simulink model "Ecotron"  (R2019b)
settings: Solver=FixedStepAuto  StartTime=0.0  StopTime=1  FixedStep=0.001  RelTol=1e-3  EnableMultiTasking=on
InitFcn:
  | EcoCoder_PreCheckLic();
libraries: CoderSF_BSW_Libs x228, SF_CanService_Libs x49, simulink x33, dspstat3 x6
(part 4 of 6)

== system Ecotron/Input/By-wire/PDS/Subsystem2 ==
  Bus Creator4 : BusCreator  Inputs=5
  Bus Creator5 : BusCreator  Inputs=4  OutDataTypeStr=Bus: Msg
      settings: InheritFromInputs=off
  Read CAN Message3 : SF_CanService_Libs/Read CAN Message  typeCAN=Connected  channel=CAN_C  mEn=off  msgInfo=ld_pds  msgItermStore=PDS_Current2Master  msgIterm=PDS_Current2Master  valid=on  stale=on  motoBit=off  setSignalName=on  flgCustomMonitorVariableRules=on  defineSignalName=off  prefixSignal='rx'  flgValTest=off  flgNoFixed=on  tSample=Task_L1ms  modeCode=Parameterless
  Subsystem1 : Subsystem
  Write and Read Measurement : CoderSF_BSW_Libs/Calibration & Measurement/Write and Read Measurement  variable_name=PDS_CH5Current  variable_value=0  variable_type=single  numD=1  unitStr=""  descStr=""
      settings: AttributesFormatString=type:%<variable_type> Dimensions:%<numD>  SourceProductName=EcoCoder Blocks
  Write and Read Measurement1 : CoderSF_BSW_Libs/Calibration & Measurement/Write and Read Measurement  variable_name=PDS_CH6Current  variable_value=0  variable_type=single  numD=1  unitStr=""  descStr=""
      settings: AttributesFormatString=type:%<variable_type> Dimensions:%<numD>  SourceProductName=EcoCoder Blocks
  Write and Read Measurement2 : CoderSF_BSW_Libs/Calibration & Measurement/Write and Read Measurement  variable_name=PDS_CH7Current  variable_value=0  variable_type=single  numD=1  unitStr=""  descStr=""
      settings: AttributesFormatString=type:%<variable_type> Dimensions:%<numD>  SourceProductName=EcoCoder Blocks
  Write and Read Measurement3 : CoderSF_BSW_Libs/Calibration & Measurement/Write and Read Measurement  variable_name=PDS_CH8Current  variable_value=0  variable_type=single  numD=1  unitStr=""  descStr=""
      settings: AttributesFormatString=type:%<variable_type> Dimensions:%<numD>  SourceProductName=EcoCoder Blocks
  Current2 : Outport
  wires:
  Read CAN Message3/2 -> Subsystem1/2(Msg_cnt)
  Read CAN Message3/1 -> Subsystem1/1("Available_in ")
  Bus Creator5/1 -> Bus Creator4/1  "Msg"
  Read CAN Message3/4 -> Write and Read Measurement1/1  "rxCURRENT6"
  Subsystem1/4(Msg_Freq) -> Bus Creator5/4  "Freq"
  Subsystem1/1("Available ") -> Bus Creator5/1  "Available"
  Subsystem1/3(Timeout_Err) -> Bus Creator5/3  "Timeout"
  Subsystem1/2(Cnt) -> Bus Creator5/2  "Cnt"
  Read CAN Message3/3 -> Write and Read Measurement/1  "rxCURRENT5"
  Read CAN Message3/6 -> Write and Read Measurement3/1  "rxCURRENT8"
  Read CAN Message3/5 -> Write and Read Measurement2/1  "rxCURRENT7"
  Bus Creator4/1 -> Current2/1  "Current2"
  Write and Read Measurement/1 -> Bus Creator4/2  "PDS_CH5Current"
  Write and Read Measurement1/1 -> Bus Creator4/3  "PDS_CH6Current"
  Write and Read Measurement2/1 -> Bus Creator4/4  "PDS_CH7Current"
  Write and Read Measurement3/1 -> Bus Creator4/5  "PDS_CH8Current"

== system Ecotron/Input/By-wire/PDS/Subsystem3 ==
  Bus Creator10 : BusCreator  Inputs=5
  Bus Creator3 : BusCreator  Inputs=4  OutDataTypeStr=Bus: Msg
      settings: InheritFromInputs=off
  Read CAN Message2 : SF_CanService_Libs/Read CAN Message  typeCAN=Connected  channel=CAN_C  mEn=off  msgInfo=ld_pds  msgItermStore=PDS_Current1Master  msgIterm=PDS_Current1Master  valid=on  stale=on  motoBit=off  setSignalName=on  flgCustomMonitorVariableRules=on  defineSignalName=off  prefixSignal='rx'  flgValTest=off  flgNoFixed=on  tSample=Task_L1ms  modeCode=Parameterless
  Subsystem2 : Subsystem
  Write and Read Measurement : CoderSF_BSW_Libs/Calibration & Measurement/Write and Read Measurement  variable_name=PDS_CH1Current  variable_value=0  variable_type=single  numD=1  unitStr=""  descStr=""
      settings: AttributesFormatString=type:%<variable_type> Dimensions:%<numD>  SourceProductName=EcoCoder Blocks
  Write and Read Measurement1 : CoderSF_BSW_Libs/Calibration & Measurement/Write and Read Measurement  variable_name=PDS_CH2Current  variable_value=0  variable_type=single  numD=1  unitStr=""  descStr=""
      settings: AttributesFormatString=type:%<variable_type> Dimensions:%<numD>  SourceProductName=EcoCoder Blocks
  Write and Read Measurement2 : CoderSF_BSW_Libs/Calibration & Measurement/Write and Read Measurement  variable_name=PDS_CH3Current  variable_value=0  variable_type=single  numD=1  unitStr=""  descStr=""
      settings: AttributesFormatString=type:%<variable_type> Dimensions:%<numD>  SourceProductName=EcoCoder Blocks
  Write and Read Measurement3 : CoderSF_BSW_Libs/Calibration & Measurement/Write and Read Measurement  variable_name=PDS_CH4Current  variable_value=0  variable_type=single  numD=1  unitStr=""  descStr=""
      settings: AttributesFormatString=type:%<variable_type> Dimensions:%<numD>  SourceProductName=EcoCoder Blocks
  Current1 : Outport
  wires:
  Subsystem2/4(Msg_Freq) -> Bus Creator3/4  "MsgFreq"
  Read CAN Message2/1 -> Subsystem2/1("Available_in ")
  Subsystem2/1("Available ") -> Bus Creator3/1  "Available"
  Subsystem2/3(Timeout_Err) -> Bus Creator3/3  "Timeout"
  Bus Creator3/1 -> Bus Creator10/1  "Msg"
  Read CAN Message2/2 -> Subsystem2/2(Msg_cnt)
  Subsystem2/2(Cnt) -> Bus Creator3/2  "Cnt"
  Read CAN Message2/5 -> Write and Read Measurement2/1  "rxCURRENT3"
  Read CAN Message2/4 -> Write and Read Measurement1/1  "rxCURRENT2"
  Read CAN Message2/3 -> Write and Read Measurement/1  "rxCURRENT1"
  Read CAN Message2/6 -> Write and Read Measurement3/1  "rxCURRENT4"
  Bus Creator10/1 -> Current1/1  "Current1"
  Write and Read Measurement/1 -> Bus Creator10/2  "PDS_CH1Current"
  Write and Read Measurement1/1 -> Bus Creator10/3  "PDS_CH2Current"
  Write and Read Measurement2/1 -> Bus Creator10/4  "PDS_CH3Current"
  Write and Read Measurement3/1 -> Bus Creator10/5  "PDS_CH4Current"

== system Ecotron/Input/By-wire/PDS/Subsystem4 ==
  Bus Creator2 : BusCreator  Inputs=4  OutDataTypeStr=Bus: Msg
      settings: InheritFromInputs=off
  Bus Creator9 : BusCreator  Inputs=4
  Read CAN Message1 : SF_CanService_Libs/Read CAN Message  typeCAN=Connected  channel=CAN_C  mEn=off  msgInfo=ld_pds  msgItermStore=PDS_Status2_Master  msgIterm=PDS_Status2_Master  valid=on  stale=on  motoBit=off  setSignalName=on  flgCustomMonitorVariableRules=on  defineSignalName=off  prefixSignal='rx'  flgValTest=off  flgNoFixed=on  tSample=Task_L1ms  modeCode=Parameterless
  Subsystem3 : Subsystem
  Write and Read Measurement : CoderSF_BSW_Libs/Calibration & Measurement/Write and Read Measurement  variable_name=PDS_BoardTemp  variable_value=0  variable_type=single  numD=1  unitStr=""  descStr=""
      settings: AttributesFormatString=type:%<variable_type> Dimensions:%<numD>  SourceProductName=EcoCoder Blocks
  Write and Read Measurement1 : CoderSF_BSW_Libs/Calibration & Measurement/Write and Read Measurement  variable_name=PDS_InputVoltage  variable_value=0  variable_type=single  numD=1  unitStr=""  descStr=""
      settings: AttributesFormatString=type:%<variable_type> Dimensions:%<numD>  SourceProductName=EcoCoder Blocks
  Write and Read Measurement2 : CoderSF_BSW_Libs/Calibration & Measurement/Write and Read Measurement  variable_name=PDS_InputCurrent  variable_value=0  variable_type=single  numD=1  unitStr=""  descStr=""
      settings: AttributesFormatString=type:%<variable_type> Dimensions:%<numD>  SourceProductName=EcoCoder Blocks
  Status2 : Outport
  wires:
  Bus Creator2/1 -> Bus Creator9/1  "Msg"
  Read CAN Message1/2 -> Subsystem3/2(Msg_cnt)
  Subsystem3/3(Timeout_Err) -> Bus Creator2/3  "Timeout"
  Subsystem3/4(Msg_Freq) -> Bus Creator2/4  "MsgFreq"
  Read CAN Message1/5 -> Write and Read Measurement2/1  "rxINPUT_CURRENT"
  Subsystem3/2(Cnt) -> Bus Creator2/2  "Cnt"
  Read CAN Message1/1 -> Subsystem3/1("Available_in ")
  Subsystem3/1("Available ") -> Bus Creator2/1  "Available"
  Read CAN Message1/4 -> Write and Read Measurement1/1  "rxINPUT_Voltage"
  Read CAN Message1/3 -> Write and Read Measurement/1  "rxBOARDTEMP"
  Bus Creator9/1 -> Status2/1  "Status2"
  Write and Read Measurement/1 -> Bus Creator9/2  "PDS_BoardTemp"
  Write and Read Measurement1/1 -> Bus Creator9/3  "PDS_InputVoltage"
  Write and Read Measurement2/1 -> Bus Creator9/4  "PDS_InputCurrent"

== system Ecotron/Input/By-wire/PDS/Subsystem6 ==
  Bus Creator11 : BusCreator  Inputs=4  OutDataTypeStr=Bus: Msg
      settings: InheritFromInputs=off
  Bus Creator12 : BusCreator  Inputs=5
  Read CAN Message5 : SF_CanService_Libs/Read CAN Message  typeCAN=Connected  channel=CAN_C  mEn=off  msgInfo=ld_pds  msgItermStore=PDS_UniteChannelStatus  msgIterm=PDS_UniteChannelStatus  valid=on  stale=on  motoBit=off  setSignalName=on  flgCustomMonitorVariableRules=on  defineSignalName=off  prefixSignal='rx'  flgValTest=off  flgNoFixed=on  tSample=Task_L1ms  modeCode=Parameterless
  Subsystem5 : Subsystem
  UnitedChannels : Outport
  wires:
  Read CAN Message5/2 -> Subsystem5/2(Msg_cnt)
  Bus Creator11/1 -> Bus Creator12/1  "Msg"
  Subsystem5/1("Available ") -> Bus Creator11/1  "Available"
  Subsystem5/4(Msg_Freq) -> Bus Creator11/4  "Freq"
  Read CAN Message5/1 -> Subsystem5/1("Available_in ")
  Read CAN Message5/3 -> Bus Creator12/2  "rxParallel_Group1"
  Subsystem5/2(Cnt) -> Bus Creator11/2  "Cnt"
  Read CAN Message5/5 -> Bus Creator12/4  "rxParallel_Group3"
  Subsystem5/3(Timeout_Err) -> Bus Creator11/3  "Timeout"
  Read CAN Message5/4 -> Bus Creator12/3  "rxParallel_Group2"
  Read CAN Message5/6 -> Bus Creator12/5  "rxParallel_Group4"
  Bus Creator12/1 -> UnitedChannels/1  "UnitedChannels"

== system Ecotron/Input/By-wire/Robeff Brake ECU/Robeff Brake FbMsg1 ==
  Bus Creator : BusCreator  Inputs=3
  Bus Creator1 : BusCreator  Inputs=4  OutDataTypeStr=Bus: Msg
      settings: InheritFromInputs=off
  Read CAN Message2 : SF_CanService_Libs/Read CAN Message  typeCAN=Connected  channel=CAN_C  mEn=off  msgInfo=RBF_DBW40_brake  msgItermStore=FeedbackMsg1  msgIterm=FeedbackMsg1  valid=on  stale=on  motoBit=off  setSignalName=on  flgCustomMonitorVariableRules=on  defineSignalName=off  prefixSignal='RBF_'  flgValTest=off  flgNoFixed=on  tSample=Task_L1ms  modeCode=Parameterless
  Subsystem4 : Subsystem
  Write and Read Measurement : CoderSF_BSW_Libs/Calibration & Measurement/Write and Read Measurement  variable_name=BBW_BrakePos  variable_value=0  variable_type=single  numD=1  unitStr=""  descStr=""
      settings: AttributesFormatString=type:%<variable_type> Dimensions:%<numD>  SourceProductName=EcoCoder Blocks
  Write and Read Measurement1 : CoderSF_BSW_Libs/Calibration & Measurement/Write and Read Measurement  variable_name=BBW_ReferenceBrakePos  variable_value=0  variable_type=single  numD=1  unitStr=""  descStr=""
      settings: AttributesFormatString=type:%<variable_type> Dimensions:%<numD>  SourceProductName=EcoCoder Blocks
  Msg1 : Outport
  wires:
  Read CAN Message2/3 -> Write and Read Measurement1/1  "RBF_ReferenceSteeringAngle"
  Bus Creator1/1 -> Bus Creator/1  "Msg"
  Read CAN Message2/2 -> Subsystem4/2(Msg_cnt)
  Read CAN Message2/1 -> Subsystem4/1("Available_in ")
  Subsystem4/1("Available ") -> Bus Creator1/1  "Available"
  Subsystem4/3(Timeout_Err) -> Bus Creator1/3  "Timeout"
  Subsystem4/4(Msg_Freq) -> Bus Creator1/4  "MsgFreq"
  Subsystem4/2(Cnt) -> Bus Creator1/2  "Cnt"
  Bus Creator/1 -> Msg1/1
  Read CAN Message2/4 -> Write and Read Measurement/1  "RBF_ActualSteeringAngle"
  Write and Read Measurement/1 -> Bus Creator/3  "BBW_BrakePos"
  Write and Read Measurement1/1 -> Bus Creator/2  "BBW_ReferenceBrakePos"

== system Ecotron/Input/By-wire/Robeff Brake ECU/Robeff Brake FbMsg2 ==
  Bus Creator : BusCreator  Inputs=7
  Bus Creator1 : BusCreator  Inputs=4  OutDataTypeStr=Bus: Msg
      settings: InheritFromInputs=off
  Read CAN Message3 : SF_CanService_Libs/Read CAN Message  typeCAN=Connected  channel=CAN_C  mEn=off  msgInfo=RBF_DBW40_brake  msgItermStore=FeedbackMsg2  msgIterm=FeedbackMsg2  valid=on  stale=on  motoBit=off  setSignalName=on  flgCustomMonitorVariableRules=on  defineSignalName=off  prefixSignal='RBF_'  flgValTest=off  flgNoFixed=on  tSample=Task_L1ms  modeCode=Parameterless
  Subsystem4 : Subsystem
  Write and Read Measurement : CoderSF_BSW_Libs/Calibration & Measurement/Write and Read Measurement  variable_name=BBW_MotorDuty  variable_value=0  variable_type=single  numD=1  unitStr=""  descStr=""
      settings: AttributesFormatString=type:%<variable_type> Dimensions:%<numD>  SourceProductName=EcoCoder Blocks
  Write and Read Measurement1 : CoderSF_BSW_Libs/Calibration & Measurement/Write and Read Measurement  variable_name=BBW_MotorCurrent  variable_value=0  variable_type=single  numD=1  unitStr=""  descStr=""
      settings: AttributesFormatString=type:%<variable_type> Dimensions:%<numD>  SourceProductName=EcoCoder Blocks
  Write and Read Measurement2 : CoderSF_BSW_Libs/Calibration & Measurement/Write and Read Measurement  variable_name=BBW_MotorVoltage  variable_value=0  variable_type=single  numD=1  unitStr=""  descStr=""
      settings: AttributesFormatString=type:%<variable_type> Dimensions:%<numD>  SourceProductName=EcoCoder Blocks
  Write and Read Measurement3 : CoderSF_BSW_Libs/Calibration & Measurement/Write and Read Measurement  variable_name=BBW_BoxTemp  variable_value=0  variable_type=single  numD=1  unitStr=""  descStr=""
      settings: AttributesFormatString=type:%<variable_type> Dimensions:%<numD>  SourceProductName=EcoCoder Blocks
  Write and Read Measurement5 : CoderSF_BSW_Libs/Calibration & Measurement/Write and Read Measurement  variable_name=BBW_RawTorqueA  variable_value=0  variable_type=single  numD=1  unitStr=""  descStr=""
      settings: AttributesFormatString=type:%<variable_type> Dimensions:%<numD>  SourceProductName=EcoCoder Blocks
  Write and Read Measurement6 : CoderSF_BSW_Libs/Calibration & Measurement/Write and Read Measurement  variable_name=BBW_RawTorqueB  variable_value=0  variable_type=single  numD=1  unitStr=""  descStr=""
      settings: AttributesFormatString=type:%<variable_type> Dimensions:%<numD>  SourceProductName=EcoCoder Blocks
  Msg2 : Outport
  wires:
  Read CAN Message3/4 -> Write and Read Measurement1/1  "RBF_MotorCurrent"
  Read CAN Message3/3 -> Write and Read Measurement/1  "RBF_MotorDuty"
  Bus Creator1/1 -> Bus Creator/1  "Msg"
  Read CAN Message3/2 -> Subsystem4/2(Msg_cnt)
  Read CAN Message3/1 -> Subsystem4/1("Available_in ")
  Subsystem4/1("Available ") -> Bus Creator1/1  "Available"
  Subsystem4/3(Timeout_Err) -> Bus Creator1/3  "Timeout"
  Subsystem4/4(Msg_Freq) -> Bus Creator1/4  "MsgFreq"
  Subsystem4/2(Cnt) -> Bus Creator1/2  "Cnt"
  Bus Creator/1 -> Msg2/1
  Read CAN Message3/5 -> Write and Read Measurement2/1  "RBF_MotorVoltage"
  Read CAN Message3/6 -> Write and Read Measurement3/1  "RBF_BoxTemperature"
  Read CAN Message3/7 -> Write and Read Measurement5/1  "RBF_RawTorqueA"
  Read CAN Message3/8 -> Write and Read Measurement6/1  "RBF_RawTorqueB"
  Write and Read Measurement/1 -> Bus Creator/2  "BBW_MotorDuty"
  Write and Read Measurement1/1 -> Bus Creator/3  "BBW_MotorCurrent"
  Write and Read Measurement2/1 -> Bus Creator/4  "BBW_MotorVoltage"
  Write and Read Measurement3/1 -> Bus Creator/5  "BBW_BoxTemp"
  Write and Read Measurement5/1 -> Bus Creator/6  "BBW_RawTorqueA"
  Write and Read Measurement6/1 -> Bus Creator/7  "BBW_RawTorqueB"

== system Ecotron/Input/By-wire/Robeff Brake ECU/Robeff Brake FbMsg3 ==
  Bus Creator : BusCreator  Inputs=9
  Bus Creator1 : BusCreator  Inputs=4  OutDataTypeStr=Bus: Msg
      settings: InheritFromInputs=off
  Read CAN Message3 : SF_CanService_Libs/Read CAN Message  typeCAN=Connected  channel=CAN_C  mEn=off  msgInfo=RBF_DBW40_brake  msgItermStore=FeedbackMsg3  msgIterm=FeedbackMsg3  valid=on  stale=on  motoBit=off  setSignalName=on  flgCustomMonitorVariableRules=on  defineSignalName=off  prefixSignal='RBF_'  flgValTest=off  flgNoFixed=on  tSample=Task_L1ms  modeCode=Parameterless
  Subsystem4 : Subsystem
  Write and Read Measurement : CoderSF_BSW_Libs/Calibration & Measurement/Write and Read Measurement  variable_name=BBW_DriverIntervention  variable_value=0  variable_type=boolean  numD=1  unitStr=""  descStr=""
      settings: AttributesFormatString=type:%<variable_type> Dimensions:%<numD>  SourceProductName=EcoCoder Blocks
  Write and Read Measurement1 : CoderSF_BSW_Libs/Calibration & Measurement/Write and Read Measurement  variable_name=BBW_CalibrationErr  variable_value=0  variable_type=boolean  numD=1  unitStr=""  descStr=""
      settings: AttributesFormatString=type:%<variable_type> Dimensions:%<numD>  SourceProductName=EcoCoder Blocks
  Write and Read Measurement2 : CoderSF_BSW_Libs/Calibration & Measurement/Write and Read Measurement  variable_name=BBW_MotorConnection  variable_value=0  variable_type=boolean  numD=1  unitStr=""  descStr=""
      settings: AttributesFormatString=type:%<variable_type> Dimensions:%<numD>  SourceProductName=EcoCoder Blocks
  Write and Read Measurement3 : CoderSF_BSW_Libs/Calibration & Measurement/Write and Read Measurement  variable_name=BBW_OverCurrent  variable_value=0  variable_type=boolean  numD=1  unitStr=""  descStr=""
      settings: AttributesFormatString=type:%<variable_type> Dimensions:%<numD>  SourceProductName=EcoCoder Blocks
  Write and Read Measurement4 : CoderSF_BSW_Libs/Calibration & Measurement/Write and Read Measurement  variable_name=BBW_AngleSensorConnection  variable_value=0  variable_type=boolean  numD=1  unitStr=""  descStr=""
      settings: AttributesFormatString=type:%<variable_type> Dimensions:%<numD>  SourceProductName=EcoCoder Blocks
  Write and Read Measurement5 : CoderSF_BSW_Libs/Calibration & Measurement/Write and Read Measurement  variable_name=BBW_ECUReset  variable_value=0  variable_type=boolean  numD=1  unitStr=""  descStr=""
      settings: AttributesFormatString=type:%<variable_type> Dimensions:%<numD>  SourceProductName=EcoCoder Blocks
  Write and Read Measurement6 : CoderSF_BSW_Libs/Calibration & Measurement/Write and Read Measurement  variable_name=BBW_UnderVoltage  variable_value=0  variable_type=boolean  numD=1  unitStr=""  descStr=""
      settings: AttributesFormatString=type:%<variable_type> Dimensions:%<numD>  SourceProductName=EcoCoder Blocks
  Write and Read Measurement7 : CoderSF_BSW_Libs/Calibration & Measurement/Write and Read Measurement  variable_name=BBW_OnCalibration  variable_value=0  variable_type=boolean  numD=1  unitStr=""  descStr=""
      settings: AttributesFormatString=type:%<variable_type> Dimensions:%<numD>  SourceProductName=EcoCoder Blocks
  "Msg3 " : Outport
  wires:
  Bus Creator1/1 -> Bus Creator/1  "Msg"
  Read CAN Message3/2 -> Subsystem4/2(Msg_cnt)
  Read CAN Message3/1 -> Subsystem4/1("Available_in ")
  Subsystem4/1("Available ") -> Bus Creator1/1  "Available"
  Subsystem4/3(Timeout_Err) -> Bus Creator1/3  "Timeout"
  Subsystem4/4(Msg_Freq) -> Bus Creator1/4  "MsgFreq"
  Subsystem4/2(Cnt) -> Bus Creator1/2  "Cnt"
  Read CAN Message3/8 -> Write and Read Measurement6/1  "RBF_UnderVoltage"
  Read CAN Message3/7 -> Write and Read Measurement5/1  "RBF_EcuReset"
  Read CAN Message3/3 -> Write and Read Measurement2/1  "RBF_MotorConnection"
  Read CAN Message3/4 -> Write and Read Measurement3/1  "RBF_OverCurrent"
  Read CAN Message3/6 -> Write and Read Measurement/1  "RBF_DriverIntervention"
  Read CAN Message3/5 -> Write and Read Measurement4/1  "RBF_AngleSensorConnection"
  Bus Creator/1 -> "Msg3 "/1
  Write and Read Measurement/1 -> Bus Creator/5  "BBW_DriverIntervention"
  Write and Read Measurement2/1 -> Bus Creator/2  "BBW_MotorConnection"
  Write and Read Measurement3/1 -> Bus Creator/3  "BBW_OverCurrent"
  Write and Read Measurement4/1 -> Bus Creator/4  "BBW_AngleSensorConnection"
  Write and Read Measurement5/1 -> Bus Creator/6  "BBW_ECUReset"
  Write and Read Measurement6/1 -> Bus Creator/7  "BBW_UnderVoltage"
  Read CAN Message3/9 -> Write and Read Measurement1/1  "RBF_CalibrationStatus"
  Read CAN Message3/10 -> Write and Read Measurement7/1  "RBF_CalibCommand_feedback"
  Write and Read Measurement1/1 -> Bus Creator/8  "BBW_CalibrationErr"
  Write and Read Measurement7/1 -> Bus Creator/9  "BBW_OnCalibration"

== system Ecotron/Input/By-wire/Robeff EPAS ECU/Robeff EPAS FbMsg1 ==
  Bus Creator : BusCreator  Inputs=3
  Bus Creator1 : BusCreator  Inputs=4  OutDataTypeStr=Bus: Msg
      settings: InheritFromInputs=off
  Read CAN Message2 : SF_CanService_Libs/Read CAN Message  typeCAN=Connected  channel=CAN_C  mEn=off  msgInfo=RBF_DBW40_speedlimit  msgItermStore=FeedbackMsg1  msgIterm=FeedbackMsg1  valid=on  stale=on  motoBit=off  setSignalName=on  flgCustomMonitorVariableRules=on  defineSignalName=off  prefixSignal='RBF_'  flgValTest=off  flgNoFixed=on  tSample=Task_L1ms  modeCode=Parameterless
  Subsystem4 : Subsystem
  Write and Read Measurement : CoderSF_BSW_Libs/Calibration & Measurement/Write and Read Measurement  variable_name=EPAS_RefSteerPos  variable_value=0  variable_type=single  numD=1  unitStr=""  descStr=""
      settings: AttributesFormatString=type:%<variable_type> Dimensions:%<numD>  SourceProductName=EcoCoder Blocks
  Write and Read Measurement1 : CoderSF_BSW_Libs/Calibration & Measurement/Write and Read Measurement  variable_name=EPAS_ActualSteeringPos  variable_value=0  variable_type=single  numD=1  unitStr=""  descStr=""
      settings: AttributesFormatString=type:%<variable_type> Dimensions:%<numD>  SourceProductName=EcoCoder Blocks
  Msg1 : Outport
  wires:
  Bus Creator/1 -> Msg1/1
  Subsystem4/2(Cnt) -> Bus Creator1/2  "Cnt"
  Subsystem4/4(Msg_Freq) -> Bus Creator1/4  "MsgFreq"
  Subsystem4/3(Timeout_Err) -> Bus Creator1/3  "Timeout"
  Subsystem4/1("Available ") -> Bus Creator1/1  "Available"
  Read CAN Message2/1 -> Subsystem4/1("Available_in ")
  Read CAN Message2/2 -> Subsystem4/2(Msg_cnt)
  Bus Creator1/1 -> Bus Creator/1  "Msg"
  Read CAN Message2/3 -> Write and Read Measurement/1  "RBF_ReferenceSteeringAngle"
  Read CAN Message2/4 -> Write and Read Measurement1/1  "RBF_ActualSteeringAngle"
  Write and Read Measurement1/1 -> Bus Creator/3  "EPAS_ActualSteeringPos"
  Write and Read Measurement/1 -> Bus Creator/2  "EPAS_RefSteerPos"

== system Ecotron/Input/By-wire/Robeff EPAS ECU/Robeff EPAS FbMsg2 ==
  Bus Creator : BusCreator  Inputs=7
  Bus Creator1 : BusCreator  Inputs=4  OutDataTypeStr=Bus: Msg
      settings: InheritFromInputs=off
  Read CAN Message3 : SF_CanService_Libs/Read CAN Message  typeCAN=Connected  channel=CAN_C  mEn=off  msgInfo=RBF_DBW40_speedlimit  msgItermStore=FeedbackMsg2  msgIterm=FeedbackMsg2  valid=on  stale=on  motoBit=off  setSignalName=on  flgCustomMonitorVariableRules=on  defineSignalName=off  prefixSignal='RBF_'  flgValTest=off  flgNoFixed=on  tSample=Task_L1ms  modeCode=Parameterless
  Subsystem4 : Subsystem
  Write and Read Measurement1 : CoderSF_BSW_Libs/Calibration & Measurement/Write and Read Measurement  variable_name=EPAS_MotorDuty  variable_value=0  variable_type=single  numD=1  unitStr=""  descStr=""
      settings: AttributesFormatString=type:%<variable_type> Dimensions:%<numD>  SourceProductName=EcoCoder Blocks
  Write and Read Measurement2 : CoderSF_BSW_Libs/Calibration & Measurement/Write and Read Measurement  variable_name=EPAS_MotorCurrent  variable_value=0  variable_type=single  numD=1  unitStr=""  descStr=""
      settings: AttributesFormatString=type:%<variable_type> Dimensions:%<numD>  SourceProductName=EcoCoder Blocks
  Write and Read Measurement3 : CoderSF_BSW_Libs/Calibration & Measurement/Write and Read Measurement  variable_name=EPAS_MotorVoltage  variable_value=0  variable_type=single  numD=1  unitStr=""  descStr=""
      settings: AttributesFormatString=type:%<variable_type> Dimensions:%<numD>  SourceProductName=EcoCoder Blocks
  Write and Read Measurement4 : CoderSF_BSW_Libs/Calibration & Measurement/Write and Read Measurement  variable_name=EPAS_TorqueA  variable_value=0  variable_type=single  numD=1  unitStr=""  descStr=""
      settings: AttributesFormatString=type:%<variable_type> Dimensions:%<numD>  SourceProductName=EcoCoder Blocks
  Write and Read Measurement5 : CoderSF_BSW_Libs/Calibration & Measurement/Write and Read Measurement  variable_name=EPAS_TorqueB  variable_value=0  variable_type=single  numD=1  unitStr=""  descStr=""
      settings: AttributesFormatString=type:%<variable_type> Dimensions:%<numD>  SourceProductName=EcoCoder Blocks
  Write and Read Measurement6 : CoderSF_BSW_Libs/Calibration & Measurement/Write and Read Measurement  variable_name=EPAS_BoxTemp  variable_value=0  variable_type=single  numD=1  unitStr=""  descStr=""
      settings: AttributesFormatString=type:%<variable_type> Dimensions:%<numD>  SourceProductName=EcoCoder Blocks
  Msg2 : Outport
  wires:
  Bus Creator/1 -> Msg2/1
  Subsystem4/2(Cnt) -> Bus Creator1/2  "Cnt"
  Subsystem4/4(Msg_Freq) -> Bus Creator1/4  "MsgFreq"
  Subsystem4/3(Timeout_Err) -> Bus Creator1/3  "Timeout"
  Subsystem4/1("Available ") -> Bus Creator1/1  "Available"
  Read CAN Message3/1 -> Subsystem4/1("Available_in ")
  Read CAN Message3/2 -> Subsystem4/2(Msg_cnt)
  Bus Creator1/1 -> Bus Creator/1  "Msg"
  Read CAN Message3/3 -> Write and Read Measurement1/1  "RBF_MotorDuty"
  Read CAN Message3/4 -> Write and Read Measurement2/1  "RBF_MotorCurrent"
  Read CAN Message3/5 -> Write and Read Measurement3/1  "RBF_MotorVoltage"
  Read CAN Message3/6 -> Write and Read Measurement6/1  "RBF_BoxTemperature"
  Read CAN Message3/7 -> Write and Read Measurement4/1  "RBF_RawTorqueA"
  Read CAN Message3/8 -> Write and Read Measurement5/1  "RBF_RawTorqueB"
  Write and Read Measurement1/1 -> Bus Creator/2  "EPAS_MotorDuty"
  Write and Read Measurement2/1 -> Bus Creator/3  "EPAS_MotorCurrent"
  Write and Read Measurement3/1 -> Bus Creator/4  "EPAS_MotorVoltage"
  Write and Read Measurement4/1 -> Bus Creator/6  "EPAS_TorqueA"
  Write and Read Measurement5/1 -> Bus Creator/7  "EPAS_TorqueB"
  Write and Read Measurement6/1 -> Bus Creator/5  "EPAS_BoxTemp"

== system Ecotron/Input/By-wire/Robeff EPAS ECU/Robeff EPAS FbMsg3 ==
  " Override Probe" : CoderSF_BSW_Libs/Calibration & Measurement/ Override Probe  variableName=EPAS_DriverIntervention_override  variableValue=0  overrideValue=0  variableDataType=boolean  variableMin=[]  variableMax=[]  variableUnitStr=""  variableDescStr=""
      settings: SourceProductName=EcoCoder Blocks
  Bus Creator : BusCreator  Inputs=7
  Bus Creator1 : BusCreator  Inputs=4  OutDataTypeStr=Bus: Msg
      settings: InheritFromInputs=off
  Read CAN Message3 : SF_CanService_Libs/Read CAN Message  typeCAN=Connected  channel=CAN_C  mEn=off  msgInfo=RBF_DBW40_speedlimit  msgItermStore=FeedbackMsg3  msgIterm=FeedbackMsg3  valid=on  stale=on  motoBit=off  setSignalName=on  flgCustomMonitorVariableRules=on  defineSignalName=off  prefixSignal='RBF_'  flgValTest=off  flgNoFixed=on  tSample=Task_L1ms  modeCode=Parameterless
  Subsystem4 : Subsystem
  Terminator : Terminator
  Write and Read Measurement : CoderSF_BSW_Libs/Calibration & Measurement/Write and Read Measurement  variable_name=EPAS_MotorConnection  variable_value=0  variable_type=boolean  numD=1  unitStr=""  descStr=""
      settings: AttributesFormatString=type:%<variable_type> Dimensions:%<numD>  SourceProductName=EcoCoder Blocks
  Write and Read Measurement1 : CoderSF_BSW_Libs/Calibration & Measurement/Write and Read Measurement  variable_name=EPAS_OverCurrent  variable_value=0  variable_type=boolean  numD=1  unitStr=""  descStr=""
      settings: AttributesFormatString=type:%<variable_type> Dimensions:%<numD>  SourceProductName=EcoCoder Blocks
  Write and Read Measurement2 : CoderSF_BSW_Libs/Calibration & Measurement/Write and Read Measurement  variable_name=EPAS_AngleSensorConnection  variable_value=0  variable_type=boolean  numD=1  unitStr=""  descStr=""
      settings: AttributesFormatString=type:%<variable_type> Dimensions:%<numD>  SourceProductName=EcoCoder Blocks
  Write and Read Measurement3 : CoderSF_BSW_Libs/Calibration & Measurement/Write and Read Measurement  variable_name=EPAS_DriverIntervention  variable_value=0  variable_type=boolean  numD=1  unitStr=""  descStr=""
      settings: AttributesFormatString=type:%<variable_type> Dimensions:%<numD>  SourceProductName=EcoCoder Blocks
  Write and Read Measurement4 : CoderSF_BSW_Libs/Calibration & Measurement/Write and Read Measurement  variable_name=EPAS_ECUReset  variable_value=0  variable_type=boolean  numD=1  unitStr=""  descStr=""
      settings: AttributesFormatString=type:%<variable_type> Dimensions:%<numD>  SourceProductName=EcoCoder Blocks
  Write and Read Measurement5 : CoderSF_BSW_Libs/Calibration & Measurement/Write and Read Measurement  variable_name=EPAS_UnderVoltage  variable_value=0  variable_type=boolean  numD=1  unitStr=""  descStr=""
      settings: AttributesFormatString=type:%<variable_type> Dimensions:%<numD>  SourceProductName=EcoCoder Blocks
  "Msg3 " : Outport
  wires:
  Bus Creator/1 -> "Msg3 "/1
  Read CAN Message3/5 -> Write and Read Measurement2/1  "RBF_AngleSensorConnection"
  Read CAN Message3/6 -> Write and Read Measurement3/1  "RBF_DriverIntervention"
  Read CAN Message3/4 -> Write and Read Measurement1/1  "RBF_OverCurrent"
  Read CAN Message3/3 -> Write and Read Measurement/1  "RBF_MotorConnection"
  Read CAN Message3/7 -> Write and Read Measurement4/1  "RBF_EcuReset"
  Read CAN Message3/8 -> Write and Read Measurement5/1  "RBF_UnderVoltage"
  Subsystem4/2(Cnt) -> Bus Creator1/2  "Cnt"
  Subsystem4/4(Msg_Freq) -> Bus Creator1/4  "MsgFreq"
  Subsystem4/3(Timeout_Err) -> Bus Creator1/3  "Timeout"
  Subsystem4/1("Available ") -> Bus Creator1/1  "Available"
  Read CAN Message3/1 -> Subsystem4/1("Available_in ")
  Read CAN Message3/2 -> Subsystem4/2(Msg_cnt)
  Bus Creator1/1 -> Bus Creator/1  "Msg"
  Write and Read Measurement/1 -> Bus Creator/2  "EPAS_MotorConnection"
  Write and Read Measurement1/1 -> Bus Creator/3  "EPAS_OverCurrent"
  Write and Read Measurement2/1 -> Bus Creator/4  "EPAS_AngleSensorConnection"
  Write and Read Measurement3/1 -> " Override Probe"/1  "EPAS_DriverIntervention"
  Write and Read Measurement4/1 -> Bus Creator/6  "EPAS_ECUReset"
  Write and Read Measurement5/1 -> Bus Creator/7  "EPAS_UnderVoltage"
  Read CAN Message3/9 -> Terminator/1  "RBF_unused"
  " Override Probe"/1 -> Bus Creator/5  "EPAS_DriverIntervention_overrideOvrMsr"

== system Ecotron/Input/By-wire/Throttle Controller/Subsystem4 ==
  "Available_in " : Inport
  Msg_cnt : Inport  Port=2
  Constant : Constant  Value=3  OutDataTypeStr=single
  Data Type Conversion : DataTypeConversion  OutDataTypeStr=single
  Delay1 : Delay  InitialCondition=0  SampleTime=0.5
  Delay2 : Delay  DelayLength=6  InitialCondition=0  SampleTime=0.5
  Delay3 : Delay  DelayLength=0  InitialCondition=0  SampleTime=0.5
  Divide : Product  Inputs=*/
  Relational Operator : RelationalOperator  Operator===  OutDataTypeStr=boolean  RndMeth=Simplest
  Subtract : Sum  Inputs=+-
  "Available " : Outport
  Cnt : Outport  Port=2
  Timeout_Err : Outport  Port=3
  Msg_Freq : Outport  Port=4
  wires:
  "Available_in "/1 -> "Available "/1
  Subtract/1 -> Data Type Conversion/1
  Relational Operator/1 -> Timeout_Err/1
  Msg_cnt/1 -> Relational Operator/1, Delay3/1, Delay1/1, Delay2/1, Cnt/1
  Delay1/1 -> Relational Operator/2
  Delay2/1 -> Subtract/2
  Data Type Conversion/1 -> Divide/1
  Divide/1 -> Msg_Freq/1
  Constant/1 -> Divide/2
  Delay3/1 -> Subtract/1

== system Ecotron/Input/Golf/BCM_01/Subsystem ==
  Trigger : TriggerPort  VariantControl=Variant  PortDimensions=1
  Constant1 : Constant  Value=0  OutDataTypeStr=boolean
  Constant2 : Constant  OutDataTypeStr=boolean
  Switch : Switch  Criteria=u2 > Threshold
  Unit Delay : UnitDelay  SampleTime=-1  HasFrameUpgradeWarning=on
  Out1 : Outport
  wires:
  Constant1/1 -> Switch/1
  Constant2/1 -> Switch/3
  Switch/1 -> Out1/1, Unit Delay/1
  Unit Delay/1 -> Switch/2

== system Ecotron/Input/Golf/BCM_01/Subsystem1 ==
  "Available_in " : Inport
  Msg_cnt : Inport  Port=2
  Constant : Constant  Value=3  OutDataTypeStr=single
  Data Type Conversion : DataTypeConversion  OutDataTypeStr=single
  Delay1 : Delay  InitialCondition=0  SampleTime=0.5
  Delay2 : Delay  DelayLength=6  InitialCondition=0  SampleTime=0.5
  Delay3 : Delay  DelayLength=0  InitialCondition=0  SampleTime=0.5
  Divide : Product  Inputs=*/
  Relational Operator : RelationalOperator  Operator===  OutDataTypeStr=boolean  RndMeth=Simplest
  Subtract : Sum  Inputs=+-
  "Available " : Outport
  Cnt : Outport  Port=2
  Timeout_Err : Outport  Port=3
  Msg_Freq : Outport  Port=4
  wires:
  Delay3/1 -> Subtract/1
  Constant/1 -> Divide/2
  Divide/1 -> Msg_Freq/1
  Data Type Conversion/1 -> Divide/1
  Delay2/1 -> Subtract/2
  Delay1/1 -> Relational Operator/2
  Msg_cnt/1 -> Cnt/1, Delay2/1, Delay1/1, Delay3/1, Relational Operator/1
  Relational Operator/1 -> Timeout_Err/1
  Subtract/1 -> Data Type Conversion/1
  "Available_in "/1 -> "Available "/1

== system Ecotron/Input/Golf/Brake/Subsystem1 ==
  "Available_in " : Inport
  Msg_cnt : Inport  Port=2
  Constant : Constant  Value=3  OutDataTypeStr=single
  Data Type Conversion : DataTypeConversion  OutDataTypeStr=single
  Delay1 : Delay  InitialCondition=0  SampleTime=0.5
  Delay2 : Delay  DelayLength=6  InitialCondition=0  SampleTime=0.5
  Delay3 : Delay  DelayLength=0  InitialCondition=0  SampleTime=0.5
  Divide : Product  Inputs=*/
  Relational Operator : RelationalOperator  Operator===  OutDataTypeStr=boolean  RndMeth=Simplest
  Subtract : Sum  Inputs=+-
  "Available " : Outport
  Cnt : Outport  Port=2
  Timeout_Err : Outport  Port=3
  Msg_Freq : Outport  Port=4
  wires:
  Delay3/1 -> Subtract/1
  Constant/1 -> Divide/2
  Divide/1 -> Msg_Freq/1
  Data Type Conversion/1 -> Divide/1
  Delay2/1 -> Subtract/2
  Delay1/1 -> Relational Operator/2
  Msg_cnt/1 -> Cnt/1, Delay2/1, Delay1/1, Delay3/1, Relational Operator/1
  Relational Operator/1 -> Timeout_Err/1
  Subtract/1 -> Data Type Conversion/1
  "Available_in "/1 -> "Available "/1

== system Ecotron/Input/Golf/Brake and Steering Feedback Echo/Subsystem2 ==
  In1 : Inport
  Trigger : TriggerPort  VariantControl=Variant  PortDimensions=1
  Send CAN Data : CoderSF_BSW_Libs/CAN/Send CAN Data  channel=CAN_C  txlen=8  txid=hex2dec('176')  frametype=Standard(11-bit ID)  showerror=off
      settings: SourceProductName=EcoCoder Blocks
  wires:
  In1/1 -> Send CAN Data/1

== system Ecotron/Input/Golf/Brake and Steering Feedback Echo/Subsystem7 ==
  In1 : Inport
  Trigger : TriggerPort  VariantControl=Variant  PortDimensions=1
  Send CAN Data : CoderSF_BSW_Libs/CAN/Send CAN Data  channel=CAN_C  txlen=8  txid=hex2dec('86')  frametype=Standard(11-bit ID)  showerror=off
      settings: SourceProductName=EcoCoder Blocks
  wires:
  In1/1 -> Send CAN Data/1

== system Ecotron/Input/Golf/EPB_01/Subsystem1 ==
  "Available_in " : Inport
  Msg_cnt : Inport  Port=2
  Constant : Constant  Value=3  OutDataTypeStr=single
  Data Type Conversion : DataTypeConversion  OutDataTypeStr=single
  Delay1 : Delay  InitialCondition=0  SampleTime=0.5
  Delay2 : Delay  DelayLength=6  InitialCondition=0  SampleTime=0.5
  Delay3 : Delay  DelayLength=0  InitialCondition=0  SampleTime=0.5
  Divide : Product  Inputs=*/
  Relational Operator : RelationalOperator  Operator===  OutDataTypeStr=boolean  RndMeth=Simplest
  Subtract : Sum  Inputs=+-
  "Available " : Outport
  Cnt : Outport  Port=2
  Timeout_Err : Outport  Port=3
  Msg_Freq : Outport  Port=4
  wires:
  Delay3/1 -> Subtract/1
  Constant/1 -> Divide/2
  Divide/1 -> Msg_Freq/1
  Data Type Conversion/1 -> Divide/1
  Delay2/1 -> Subtract/2
  Delay1/1 -> Relational Operator/2
  Msg_cnt/1 -> Cnt/1, Delay2/1, Delay1/1, Delay3/1, Relational Operator/1
  Relational Operator/1 -> Timeout_Err/1
  Subtract/1 -> Data Type Conversion/1
  "Available_in "/1 -> "Available "/1

== system Ecotron/Input/Golf/ESP_05/Subsystem1 ==
  "Available_in " : Inport
  Msg_cnt : Inport  Port=2
  Constant : Constant  Value=3  OutDataTypeStr=single
  Data Type Conversion : DataTypeConversion  OutDataTypeStr=single
  Delay1 : Delay  InitialCondition=0  SampleTime=0.5
  Delay2 : Delay  DelayLength=6  InitialCondition=0  SampleTime=0.5
  Delay3 : Delay  DelayLength=0  InitialCondition=0  SampleTime=0.5
  Divide : Product  Inputs=*/
  Relational Operator : RelationalOperator  Operator===  OutDataTypeStr=boolean  RndMeth=Simplest
  Subtract : Sum  Inputs=+-
  "Available " : Outport
  Cnt : Outport  Port=2
  Timeout_Err : Outport  Port=3
  Msg_Freq : Outport  Port=4
  wires:
  Delay3/1 -> Subtract/1
  Constant/1 -> Divide/2
  Divide/1 -> Msg_Freq/1
  Data Type Conversion/1 -> Divide/1
  Delay2/1 -> Subtract/2
  Delay1/1 -> Relational Operator/2
  Msg_cnt/1 -> Cnt/1, Delay2/1, Delay1/1, Delay3/1, Relational Operator/1
  Relational Operator/1 -> Timeout_Err/1
  Subtract/1 -> Data Type Conversion/1
  "Available_in "/1 -> "Available "/1

== system Ecotron/Input/Golf/Gateway_72/Subsystem1 ==
  "Available_in " : Inport
  Msg_cnt : Inport  Port=2
  Constant : Constant  Value=3  OutDataTypeStr=single
  Data Type Conversion : DataTypeConversion  OutDataTypeStr=single
  Delay1 : Delay  InitialCondition=0  SampleTime=0.5
  Delay2 : Delay  DelayLength=6  InitialCondition=0  SampleTime=0.5
  Delay3 : Delay  DelayLength=0  InitialCondition=0  SampleTime=0.5
  Divide : Product  Inputs=*/
  Relational Operator : RelationalOperator  Operator===  OutDataTypeStr=boolean  RndMeth=Simplest
  Subtract : Sum  Inputs=+-
  "Available " : Outport
  Cnt : Outport  Port=2
  Timeout_Err : Outport  Port=3
  Msg_Freq : Outport  Port=4
  wires:
  Delay3/1 -> Subtract/1
  Constant/1 -> Divide/2
  Divide/1 -> Msg_Freq/1
  Data Type Conversion/1 -> Divide/1
  Delay2/1 -> Subtract/2
  Delay1/1 -> Relational Operator/2
  Msg_cnt/1 -> Cnt/1, Delay2/1, Delay1/1, Delay3/1, Relational Operator/1
  Relational Operator/1 -> Timeout_Err/1
  Subtract/1 -> Data Type Conversion/1
  "Available_in "/1 -> "Available "/1

== system Ecotron/Input/Golf/Getriebe_1/Subsystem1 ==
  "Available_in " : Inport
  Msg_cnt : Inport  Port=2
  Constant : Constant  Value=3  OutDataTypeStr=single
  Data Type Conversion : DataTypeConversion  OutDataTypeStr=single
  Delay1 : Delay  InitialCondition=0  SampleTime=0.5
  Delay2 : Delay  DelayLength=6  InitialCondition=0  SampleTime=0.5
  Delay3 : Delay  DelayLength=0  InitialCondition=0  SampleTime=0.5
  Divide : Product  Inputs=*/
  Relational Operator : RelationalOperator  Operator===  OutDataTypeStr=boolean  RndMeth=Simplest
  Subtract : Sum  Inputs=+-
  "Available " : Outport
  Cnt : Outport  Port=2
  Timeout_Err : Outport  Port=3
  Msg_Freq : Outport  Port=4
  wires:
  Delay3/1 -> Subtract/1
  Constant/1 -> Divide/2
  Divide/1 -> Msg_Freq/1
  Data Type Conversion/1 -> Divide/1
  Delay2/1 -> Subtract/2
  Delay1/1 -> Relational Operator/2
  Msg_cnt/1 -> Cnt/1, Delay2/1, Delay1/1, Delay3/1, Relational Operator/1
  Relational Operator/1 -> Timeout_Err/1
  Subtract/1 -> Data Type Conversion/1
  "Available_in "/1 -> "Available "/1

== system Ecotron/Input/Golf/Getriebe_11/Subsystem1 ==
  "Available_in " : Inport
  Msg_cnt : Inport  Port=2
  Constant : Constant  Value=3  OutDataTypeStr=single
  Data Type Conversion : DataTypeConversion  OutDataTypeStr=single
  Delay1 : Delay  InitialCondition=0  SampleTime=0.5
  Delay2 : Delay  DelayLength=6  InitialCondition=0  SampleTime=0.5
  Delay3 : Delay  DelayLength=0  InitialCondition=0  SampleTime=0.5
  Divide : Product  Inputs=*/
  Relational Operator : RelationalOperator  Operator===  OutDataTypeStr=boolean  RndMeth=Simplest
  Subtract : Sum  Inputs=+-
  "Available " : Outport
  Cnt : Outport  Port=2
  Timeout_Err : Outport  Port=3
  Msg_Freq : Outport  Port=4
  wires:
  "Available_in "/1 -> "Available "/1
  Subtract/1 -> Data Type Conversion/1
  Relational Operator/1 -> Timeout_Err/1
  Msg_cnt/1 -> Relational Operator/1, Delay3/1, Delay1/1, Delay2/1, Cnt/1
  Delay1/1 -> Relational Operator/2
  Delay2/1 -> Subtract/2
  Data Type Conversion/1 -> Divide/1
  Divide/1 -> Msg_Freq/1
  Constant/1 -> Divide/2
  Delay3/1 -> Subtract/1

== system Ecotron/Input/Golf/Getriebe_2/Subsystem1 ==
  "Available_in " : Inport
  Msg_cnt : Inport  Port=2
  Constant : Constant  Value=3  OutDataTypeStr=single
  Data Type Conversion : DataTypeConversion  OutDataTypeStr=single
  Delay1 : Delay  InitialCondition=0  SampleTime=0.5
  Delay2 : Delay  DelayLength=6  InitialCondition=0  SampleTime=0.5
  Delay3 : Delay  DelayLength=0  InitialCondition=0  SampleTime=0.5
  Divide : Product  Inputs=*/
  Relational Operator : RelationalOperator  Operator===  OutDataTypeStr=boolean  RndMeth=Simplest
  Subtract : Sum  Inputs=+-
  "Available " : Outport
  Cnt : Outport  Port=2
  Timeout_Err : Outport  Port=3
  Msg_Freq : Outport  Port=4
  wires:
  "Available_in "/1 -> "Available "/1
  Subtract/1 -> Data Type Conversion/1
  Relational Operator/1 -> Timeout_Err/1
  Msg_cnt/1 -> Relational Operator/1, Delay3/1, Delay1/1, Delay2/1, Cnt/1
  Delay1/1 -> Relational Operator/2
  Delay2/1 -> Subtract/2
  Data Type Conversion/1 -> Divide/1
  Divide/1 -> Msg_Freq/1
  Constant/1 -> Divide/2
  Delay3/1 -> Subtract/1

== system Ecotron/Input/Golf/Kombi_02/Subsystem1 ==
  "Available_in " : Inport
  Msg_cnt : Inport  Port=2
  Constant : Constant  Value=3  OutDataTypeStr=single
  Data Type Conversion : DataTypeConversion  OutDataTypeStr=single
  Delay1 : Delay  InitialCondition=0  SampleTime=0.5
  Delay2 : Delay  DelayLength=6  InitialCondition=0  SampleTime=0.5
  Delay3 : Delay  DelayLength=0  InitialCondition=0  SampleTime=0.5
  Divide : Product  Inputs=*/
  Relational Operator : RelationalOperator  Operator===  OutDataTypeStr=boolean  RndMeth=Simplest
  Subtract : Sum  Inputs=+-
  "Available " : Outport
  Cnt : Outport  Port=2
  Timeout_Err : Outport  Port=3
  Msg_Freq : Outport  Port=4
  wires:
  "Available_in "/1 -> "Available "/1
  Subtract/1 -> Data Type Conversion/1
  Relational Operator/1 -> Timeout_Err/1
  Msg_cnt/1 -> Relational Operator/1, Delay3/1, Delay1/1, Delay2/1, Cnt/1
  Delay1/1 -> Relational Operator/2
  Delay2/1 -> Subtract/2
  Data Type Conversion/1 -> Divide/1
  Divide/1 -> Msg_Freq/1
  Constant/1 -> Divide/2
  Delay3/1 -> Subtract/1

== system Ecotron/Input/Golf/LWl/Subsystem1 ==
  "Available_in " : Inport
  Msg_cnt : Inport  Port=2
  Constant : Constant  Value=3  OutDataTypeStr=single
  Data Type Conversion : DataTypeConversion  OutDataTypeStr=single
  Delay1 : Delay  InitialCondition=0  SampleTime=0.5
  Delay2 : Delay  DelayLength=6  InitialCondition=0  SampleTime=0.5
  Delay3 : Delay  DelayLength=0  InitialCondition=0  SampleTime=0.5
  Divide : Product  Inputs=*/
  Relational Operator : RelationalOperator  Operator===  OutDataTypeStr=boolean  RndMeth=Simplest
  Subtract : Sum  Inputs=+-
  "Available " : Outport
  Cnt : Outport  Port=2
  Timeout_Err : Outport  Port=3
  Msg_Freq : Outport  Port=4
  wires:
  Delay3/1 -> Subtract/1
  Constant/1 -> Divide/2
  Divide/1 -> Msg_Freq/1
  Data Type Conversion/1 -> Divide/1
  Delay2/1 -> Subtract/2
  Delay1/1 -> Relational Operator/2
  Msg_cnt/1 -> Cnt/1, Delay2/1, Delay1/1, Delay3/1, Relational Operator/1
  Relational Operator/1 -> Timeout_Err/1
  Subtract/1 -> Data Type Conversion/1
  "Available_in "/1 -> "Available "/1

== system Ecotron/Input/Golf/Motor_11/Subsystem1 ==
  "Available_in " : Inport
  Msg_cnt : Inport  Port=2
  Constant : Constant  Value=3  OutDataTypeStr=single
  Data Type Conversion : DataTypeConversion  OutDataTypeStr=single
  Delay1 : Delay  InitialCondition=0  SampleTime=0.5
  Delay2 : Delay  DelayLength=6  InitialCondition=0  SampleTime=0.5
  Delay3 : Delay  DelayLength=0  InitialCondition=0  SampleTime=0.5
  Divide : Product  Inputs=*/
  Relational Operator : RelationalOperator  Operator===  OutDataTypeStr=boolean  RndMeth=Simplest
  Subtract : Sum  Inputs=+-
  "Available " : Outport
  Cnt : Outport  Port=2
  Timeout_Err : Outport  Port=3
  Msg_Freq : Outport  Port=4
  wires:
  Delay3/1 -> Subtract/1
  Constant/1 -> Divide/2
  Divide/1 -> Msg_Freq/1
  Data Type Conversion/1 -> Divide/1
  Delay2/1 -> Subtract/2
  Delay1/1 -> Relational Operator/2
  Msg_cnt/1 -> Cnt/1, Delay2/1, Delay1/1, Delay3/1, Relational Operator/1
  Relational Operator/1 -> Timeout_Err/1
  Subtract/1 -> Data Type Conversion/1
  "Available_in "/1 -> "Available "/1

== system Ecotron/Input/Golf/Motor_12/Subsystem1 ==
  "Available_in " : Inport
  Msg_cnt : Inport  Port=2
  Constant : Constant  Value=3  OutDataTypeStr=single
  Data Type Conversion : DataTypeConversion  OutDataTypeStr=single
  Delay1 : Delay  InitialCondition=0  SampleTime=0.5
  Delay2 : Delay  DelayLength=6  InitialCondition=0  SampleTime=0.5
  Delay3 : Delay  DelayLength=0  InitialCondition=0  SampleTime=0.5
  Divide : Product  Inputs=*/
  Relational Operator : RelationalOperator  Operator===  OutDataTypeStr=boolean  RndMeth=Simplest
  Subtract : Sum  Inputs=+-
  "Available " : Outport
  Cnt : Outport  Port=2
  Timeout_Err : Outport  Port=3
  Msg_Freq : Outport  Port=4
  wires:
  Delay3/1 -> Subtract/1
  Constant/1 -> Divide/2
  Divide/1 -> Msg_Freq/1
  Data Type Conversion/1 -> Divide/1
  Delay2/1 -> Subtract/2
  Delay1/1 -> Relational Operator/2
  Msg_cnt/1 -> Cnt/1, Delay2/1, Delay1/1, Delay3/1, Relational Operator/1
  Relational Operator/1 -> Timeout_Err/1
  Subtract/1 -> Data Type Conversion/1
  "Available_in "/1 -> "Available "/1

== system Ecotron/Input/Golf/Motor_14/Subsystem1 ==
  "Available_in " : Inport
  Msg_cnt : Inport  Port=2
  Constant : Constant  Value=3  OutDataTypeStr=single
  Data Type Conversion : DataTypeConversion  OutDataTypeStr=single
  Delay1 : Delay  InitialCondition=0  SampleTime=0.5
  Delay2 : Delay  DelayLength=6  InitialCondition=0  SampleTime=0.5
  Delay3 : Delay  DelayLength=0  InitialCondition=0  SampleTime=0.5
  Divide : Product  Inputs=*/
  Relational Operator : RelationalOperator  Operator===  OutDataTypeStr=boolean  RndMeth=Simplest
  Subtract : Sum  Inputs=+-
  "Available " : Outport
  Cnt : Outport  Port=2
  Timeout_Err : Outport  Port=3
  Msg_Freq : Outport  Port=4
  wires:
  Delay3/1 -> Subtract/1
  Constant/1 -> Divide/2
  Divide/1 -> Msg_Freq/1
  Data Type Conversion/1 -> Divide/1
  Delay2/1 -> Subtract/2
  Delay1/1 -> Relational Operator/2
  Msg_cnt/1 -> Cnt/1, Delay2/1, Delay1/1, Delay3/1, Relational Operator/1
  Relational Operator/1 -> Timeout_Err/1
  Subtract/1 -> Data Type Conversion/1
  "Available_in "/1 -> "Available "/1

== system Ecotron/Input/Golf/Motor_20/Subsystem1 ==
  "Available_in " : Inport
  Msg_cnt : Inport  Port=2
  Constant : Constant  Value=3  OutDataTypeStr=single
  Data Type Conversion : DataTypeConversion  OutDataTypeStr=single
  Delay1 : Delay  InitialCondition=0  SampleTime=0.5
  Delay2 : Delay  DelayLength=6  InitialCondition=0  SampleTime=0.5
  Delay3 : Delay  DelayLength=0  InitialCondition=0  SampleTime=0.5
  Divide : Product  Inputs=*/
  Relational Operator : RelationalOperator  Operator===  OutDataTypeStr=boolean  RndMeth=Simplest
  Subtract : Sum  Inputs=+-
  "Available " : Outport
  Cnt : Outport  Port=2
  Timeout_Err : Outport  Port=3
  Msg_Freq : Outport  Port=4
  wires:
  Delay3/1 -> Subtract/1
  Constant/1 -> Divide/2
  Divide/1 -> Msg_Freq/1
  Data Type Conversion/1 -> Divide/1
  Delay2/1 -> Subtract/2
  Delay1/1 -> Relational Operator/2
  Msg_cnt/1 -> Cnt/1, Delay2/1, Delay1/1, Delay3/1, Relational Operator/1
  Relational Operator/1 -> Timeout_Err/1
  Subtract/1 -> Data Type Conversion/1
  "Available_in "/1 -> "Available "/1

== system Ecotron/Input/Golf/Subsystem/Subsystem1 ==
  "Available_in " : Inport
  Msg_cnt : Inport  Port=2
  Constant : Constant  Value=3  OutDataTypeStr=single
  Data Type Conversion : DataTypeConversion  OutDataTypeStr=single
  Delay1 : Delay  InitialCondition=0  SampleTime=0.5
  Delay2 : Delay  DelayLength=6  InitialCondition=0  SampleTime=0.5
  Delay3 : Delay  DelayLength=0  InitialCondition=0  SampleTime=0.5
  Divide : Product  Inputs=*/
  Relational Operator : RelationalOperator  Operator===  OutDataTypeStr=boolean  RndMeth=Simplest
  Subtract : Sum  Inputs=+-
  "Available " : Outport
  Cnt : Outport  Port=2
  Timeout_Err : Outport  Port=3
  Msg_Freq : Outport  Port=4
  wires:
  Delay3/1 -> Subtract/1
  Constant/1 -> Divide/2
  Divide/1 -> Msg_Freq/1
  Data Type Conversion/1 -> Divide/1
  Delay2/1 -> Subtract/2
  Delay1/1 -> Relational Operator/2
  Msg_cnt/1 -> Cnt/1, Delay2/1, Delay1/1, Delay3/1, Relational Operator/1
  Relational Operator/1 -> Timeout_Err/1
  Subtract/1 -> Data Type Conversion/1
  "Available_in "/1 -> "Available "/1

== system Ecotron/Input/Golf/WheelSpeed/Subsystem1 ==
  "Available_in " : Inport
  Msg_cnt : Inport  Port=2
  Constant : Constant  Value=3  OutDataTypeStr=single
  Data Type Conversion : DataTypeConversion  OutDataTypeStr=single
  Delay1 : Delay  InitialCondition=0  SampleTime=0.5
  Delay2 : Delay  DelayLength=6  InitialCondition=0  SampleTime=0.5
  Delay3 : Delay  DelayLength=0  InitialCondition=0  SampleTime=0.5
  Divide : Product  Inputs=*/
  Relational Operator : RelationalOperator  Operator===  OutDataTypeStr=boolean  RndMeth=Simplest
  Subtract : Sum  Inputs=+-
  "Available " : Outport
  Cnt : Outport  Port=2
  Timeout_Err : Outport  Port=3
  Msg_Freq : Outport  Port=4
  wires:
  Delay3/1 -> Subtract/1
  Constant/1 -> Divide/2
  Divide/1 -> Msg_Freq/1
  Data Type Conversion/1 -> Divide/1
  Delay2/1 -> Subtract/2
  Delay1/1 -> Relational Operator/2
  Msg_cnt/1 -> Cnt/1, Delay2/1, Delay1/1, Delay3/1, Relational Operator/1
  Relational Operator/1 -> Timeout_Err/1
  Subtract/1 -> Data Type Conversion/1
  "Available_in "/1 -> "Available "/1
